simulink model "Receiver_Final"  (R2023b)
settings: Solver=FixedStepAuto  StartTime=0.0  StopTime=10.0  RelTol=1e-3
undefined symbols (not defined in the file): ax, ay, az, Data_Display, Data_Input, gx, gy, gz, Hasan_Receiver
libraries: androiduilib x8, androidaudiovideolib x1, androidcommunicationlib x1
settings Model: Creator=Lenovo-pc  LastModifiedBy=krish
settings OptimizationCC: EnhancedBackFolding=on  PassReuseOutputArgsAs=Individual arguments  ZeroExternalMemoryAtStartup=off  ZeroInternalMemoryAtStartup=off  MaxStackSize=64  OptimizeBlockOrder=speed  DifferentSizesBufferReuse=on  OptimizationCustomize=off  EfficientTunableParamExpr=on
settings DebuggingCC: ParameterTunabilityLossMsg=error
settings HardwareCC: ProdBitPerLong=64  ProdLargestAtomicInteger=LongLong  ProdLargestAtomicFloat=Double  ProdLongLongMode=on  ProdHWDeviceType=ARM Compatible->ARM 64-bit (LP64)  UseEmbeddedCoderFeatures=off  UseSimulinkCoderFeatures=off
settings SFSimCC: MATLABDynamicMemAlloc=off
settings RTWCC: Description=Embedded Coder  SystemTargetFile=ert.tlc  HardwareBoard=Android Device (64bit)  TLCOptions="-aInlineSetEventsForThisBaseRateFcn=TLC_FALSE -aSuppressMultiTaskScheduler=TLC_FALSE  -aRateBasedStepFcn=0"  TemplateMakefile=ert_default_tmf  RTWVerbose=off  Toolchain=Android SDK/NDK Tools
settings CodeAppCC: ForceParamTrailComments=on  IgnoreCustomStorageClasses=off  OperatorAnnotations=on  SimulinkDataObjDesc=on  SFDataObjDesc=on  InsertBlockDesc=on
settings ERTTargetCC: SupportNonInlinedSFcns=on

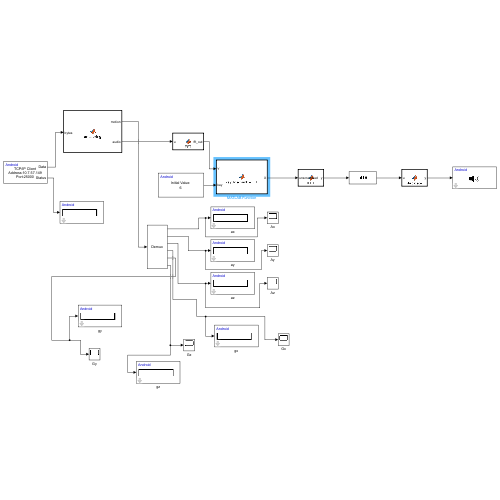
[thumbnail: Simulink's stored preview of the top-level diagram]
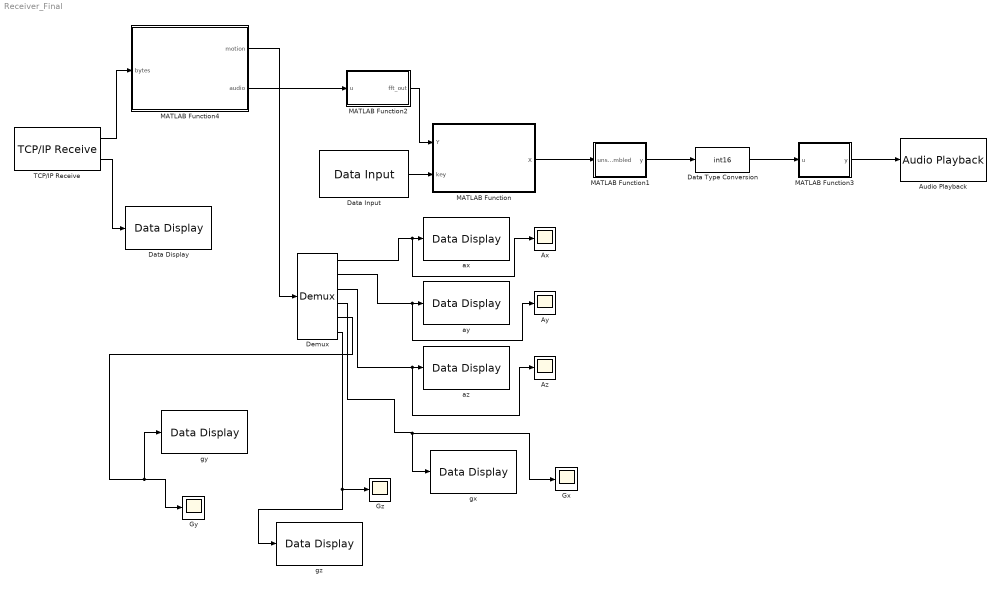
== system Receiver_Final ==
  Audio Playback : androidaudiovideolib/Audio Playback  SampleFreq=44100  AudioSamplingFreq=44100  SampleTime=0.1  DeviceStr=0  QueueDuration=0  BlockPlatform=Android
  Ax : Scope
  Ay : Scope
  Az : Scope
  Data Display : androiduilib/Data Display  DataDisplayId=Hasan_Receiver/Data_Display  Format=Float  Precision=6  SimulateUsing=Code generation  blockPlatform=Android
  Data Input : androiduilib/Data Input  isCharVector=off  Value=6  CharVector=Hello World  OutputDataType=double  maxCharVectorSize=100  DataInputId=Hasan_Receiver/Data_Input  SampleTime=0.1
  Data Type Conversion : DataTypeConversion  OutDataTypeStr=int16  SaturateOnIntegerOverflow=off  RndMeth=Floor
  Demux : Demux  Outputs=6
      settings: DisplayOption=none
  Gx : Scope
  Gy : Scope
  Gz : Scope
  MATLAB Function : MATLAB Function  TreatAsAtomicUnit=on
  MATLAB Function1 : MATLAB Function  TreatAsAtomicUnit=on
  MATLAB Function2 : MATLAB Function  TreatAsAtomicUnit=on
  MATLAB Function3 : MATLAB Function  TreatAsAtomicUnit=on
  MATLAB Function4 : MATLAB Function  TreatAsAtomicUnit=on
  TCP/IP Receive : androidcommunicationlib/TCP//IP Receive  TCPReceiveId=Hasan_Receiver/TCP//IP_Receive  Mode_=Client  LocalServerPort_=25000  RemoteAddr_=10.7.57.149  RemoteServerPort_=25000  DataType_=uint8  DataSize_=8844  SampleTime_=0.1  ClientPortBindingSelection_=off  ClientPortToBind_=35000  BlockingMode_=on  BlockTimeout_=0.1
  ax : androiduilib/Data Display  DataDisplayId=Hasan_Receiver/ax  Format=Float  Precision=6  SimulateUsing=Code generation  blockPlatform=Android
  ay : androiduilib/Data Display  DataDisplayId=Hasan_Receiver/ay  Format=Float  Precision=6  SimulateUsing=Code generation  blockPlatform=Android
  az : androiduilib/Data Display  DataDisplayId=Hasan_Receiver/az  Format=Float  Precision=6  SimulateUsing=Code generation  blockPlatform=Android
  gx : androiduilib/Data Display  DataDisplayId=Hasan_Receiver/gx  Format=Float  Precision=6  SimulateUsing=Code generation  blockPlatform=Android
  gy : androiduilib/Data Display  DataDisplayId=Hasan_Receiver/gy  Format=Float  Precision=6  SimulateUsing=Code generation  blockPlatform=Android
  gz : androiduilib/Data Display  DataDisplayId=Hasan_Receiver/gz  Format=Float  Precision=6  SimulateUsing=Code generation  blockPlatform=Android
  wires:
  MATLAB Function/1(X) -> MATLAB Function1/1(unscrambled)
  MATLAB Function2/1(fft_out) -> MATLAB Function/1(Y)
  MATLAB Function1/1(y) -> Data Type Conversion/1
  TCP/IP Receive/1 -> MATLAB Function4/1(bytes)
  Data Input/1 -> MATLAB Function/2(key)
  Demux/1 -> Ax/1, ax/1
  Demux/2 -> Ay/1, ay/1
  Demux/3 -> Az/1, az/1
  Demux/4 -> gx/1, Gx/1
  Demux/5 -> Gy/1, gy/1
  Demux/6 -> gz/1, Gz/1
  Data Type Conversion/1 -> MATLAB Function3/1(u)
  MATLAB Function4/2(audio) -> MATLAB Function2/1(u)
  MATLAB Function3/1(y) -> Audio Playback/1
  TCP/IP Receive/2 -> Data Display/1
  MATLAB Function4/1(motion) -> Demux/1

== matlab function Receiver_Final/MATLAB Function ==
  data: Y input; X output; key input
% function X = keyUnscrambleFFT(Y, key)
% 
%     [N, C] = size(Y);
% 
%     posIdx = 2:floor(N/2);
%     negIdx = N - posIdx + 2;
%     K = numel(posIdx);
%     if K == 0
%         X = Y;
%         return;
%     end
% 
% 
%     b = mod(key, K);
%     a = mod(key, K-1) + 1;
% 
%     while K > 1 && gcd(a, K) ~= 1
%         a = a + 1;
%         if a >= K
%             a = 1;
%         end
%     end
% 
%     inv_a = modInverse(a, K);
% 
%     inv_perm = zeros(1, K);
%     for m = 1:K
%         inv_perm(m) = mod(inv_a * ((m-1) - b), K) + 1;
%     end
% 
%     if ~isreal(Y)
%         X = complex(zeros(N, C, 'like', Y));
%     else
%         X = zeros(N, C, 'like', Y);
%     end
% 
%     X(1, :) = Y(1, :);
%     if mod(N, 2) == 0
%         X(N/2 + 1, :) = Y(N/2 + 1, :);
%     end
% 
%     X(posIdx, :) = Y(posIdx(inv_perm), :);
% 
%     if ~isreal(Y)
%         X(negIdx, :) = conj(X(posIdx, :));
%     else
%         X(negIdx, :) = X(posIdx, :);
%     end
% end
% 
% function inv_a = modInverse(a, K)
% 
%     [g, inv_a, ~] = gcd(a, K);
%     if g ~= 1
%         error('Modular inverse does not exist.');
%     end
%     inv_a = mod(inv_a, K);
%     if inv_a < 0
%         inv_a = inv_a + K;
%     end
% end

function X = keyUnscrambleFFT(Y, key)
    [N, C] = size(Y);

    posIdx = 2:floor(N/2);
    negIdx = N - posIdx + 2;
    K = numel(posIdx);
    % K=5;
    if K == 0
        X = Y;
        return;
    end


    b = mod(key, K);
    a = mod(key, K-1) + 1;

    while K > 1 && gcd(a, K) ~= 1
        a = a + 1;
        if a >= K
            a = 1;
        end
    end

    inv_a = modInverse(a, K);

    inv_perm = zeros(1, K);
    for m = 1:K
        inv_perm(m) = mod(inv_a * ((m-1) - b), K) + 1;
    end

    if ~isreal(Y)
        X = complex(zeros(N, C, 'like', Y));
    else
        X = zeros(N, C, 'like', Y);
    end

    X(1, :) = Y(1, :);
    if mod(N, 2) == 0
        X(N/2 + 1, :) = Y(N/2 + 1, :);
    end

    X(posIdx, :) = Y(posIdx(inv_perm), :);

    if ~isreal(Y)
        X(negIdx, :) = conj(X(posIdx, :));
    else
        X(negIdx, :) = X(posIdx, :);
    end
end

function inv_a = modInverse(a, K)
    [g, inv_a, ~] = gcd(a, K);
    if g ~= 1
        error('no modular inverse');
    end
    inv_a = mod(inv_a, K);
    if inv_a < 0
        inv_a = inv_a + K;
    end
end

== matlab function Receiver_Final/MATLAB Function2 ==
  data: u input; fft_out output
function fft_out = FFT(u)
    u = u(:,1);
    fft_out = fft(u);
end

== matlab function Receiver_Final/MATLAB Function3 ==
  data: u input; y output
function y = duplicate(u)
y = [u, u];

== matlab function Receiver_Final/MATLAB Function4 ==
  data: bytes input; motion output; audio output
function [motion, audio] = unpacking(bytes)
                 
motion = zeros(1,6,'single');         % 1x6
audio = zeros(4410,1,'int16');       % 4410x1


motion(1,1:6)  = typecast(bytes(1:24), 'single').';   % 6 singles
audio(:,1)  = typecast(bytes(25:8844), 'int16');   % 4410 samples
end

== matlab function Receiver_Final/MATLAB Function1 ==
  data: unscrambled input; y output
function y = IFFT(unscrambled)
    N = length(unscrambled);
    unscrambled(2:N/2) = conj(unscrambled(N:-1:N/2+2));
    Channel = ifft(unscrambled);
    y = real(Channel);
end
